simulink model "Platoon"  (Simulink 7.6)
settings: Solver=ode45  StartTime=0  StopTime=120  RelTol=1e-3
libraries: Solver_SF x5
settings Model: Creator=dhall  LastModifiedBy=mkhan  ExtModeTrigMode=oneshot  ExtModeArmWhenConnect=off
settings DataIOCC: LimitDataPoints=off  SignalLoggingName=sigsOut
settings OptimizationCC: BooleanDataType=off  LocalBlockOutputs=off  InitFltsAndDblsToZero=on
settings DebuggingCC: SaveWithParameterizedLinksMsg=none  SignalResolutionControl=TryResolveAllWithWarning  SolverPrmCheckMsg=none  MultiTaskDSMMsg=warning  MultiTaskCondExecSysMsg=none  FcnCallInpInsideContextMsg=Enable All
settings HardwareCC: TargetHWDeviceType=32-bit Generic  TargetUnknown=on  ProdEqTarget=off
settings CodeAppCC: CustomSymbolStrType=$N$R$M_T
settings GRTTargetCC: TargetFcnLib=ansi_tfl_tmw.mat  TargetFunctionLibrary=C89/C90 (ANSI)

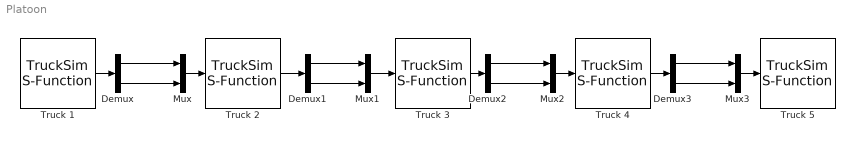
== system Platoon ==
  Demux{,1..3} (4 alike) : Demux  Outputs=2
  Mux{,1..3} (4 alike) : Mux  Inputs=2
  Truck 1 : Solver_SF/TruckSim S-Function  Priority=1  SIMFILE=Platoon_Truck_1.sim  Run_RTs=off  vs_state_ind=Run  StopMode_ind=Vehicle Model
  Truck 2 : Solver_SF/TruckSim S-Function  Priority=1  SIMFILE=Platoon_Truck_2.sim  Run_RTs=off  vs_state_ind=Run  StopMode_ind=Vehicle Model
  Truck 3 : Solver_SF/TruckSim S-Function  Priority=1  SIMFILE=Platoon_Truck_3.sim  Run_RTs=off  vs_state_ind=Run  StopMode_ind=Vehicle Model
  Truck 4 : Solver_SF/TruckSim S-Function  Priority=1  SIMFILE=Platoon_Truck_4.sim  Run_RTs=off  vs_state_ind=Run  StopMode_ind=Vehicle Model
  Truck 5 : Solver_SF/TruckSim S-Function  Priority=1  SIMFILE=Platoon_Truck_5.sim  Run_RTs=off  vs_state_ind=Run  StopMode_ind=Vehicle Model
  wires:
  Demux/2 -> Mux/2
  Demux/1 -> Mux/1
  Demux1/2 -> Mux1/2
  Demux1/1 -> Mux1/1
  Demux2/2 -> Mux2/2
  Demux2/1 -> Mux2/1
  Demux3/2 -> Mux3/2
  Demux3/1 -> Mux3/1
  Truck 1/1 -> Demux/1
  Mux/1 -> Truck 2/1
  Truck 2/1 -> Demux1/1
  Mux1/1 -> Truck 3/1
  Truck 3/1 -> Demux2/1
  Mux2/1 -> Truck 4/1
  Truck 4/1 -> Demux3/1
  Mux3/1 -> Truck 5/1
